simulink model "Non_linear_model_impulse_response"  (R2021b)
settings: Solver=FixedStepAuto  StartTime=0.0  StopTime=30  FixedStep=0.001  RelTol=1e-3  EnableMultiTasking=on
values from neighbouring files (symbols this model uses):
  F = 1.5    [Initial_data.m]
  F_j = 2.7    [Initial_data.m]
  F_js = 1.5    [Initial_data.m]
  F_s = 1    [Initial_data.m]
  T_i = 57    [Initial_data.m]
  T_is = 50    [Initial_data.m]
  T_ji = 206    [Initial_data.m]
  T_jis = 200    [Initial_data.m]
  T_js = 150    [Initial_data.m]
  T_s = 125    [Initial_data.m]
settings Model: Creator=Administrator  LastModifiedBy=Administrator

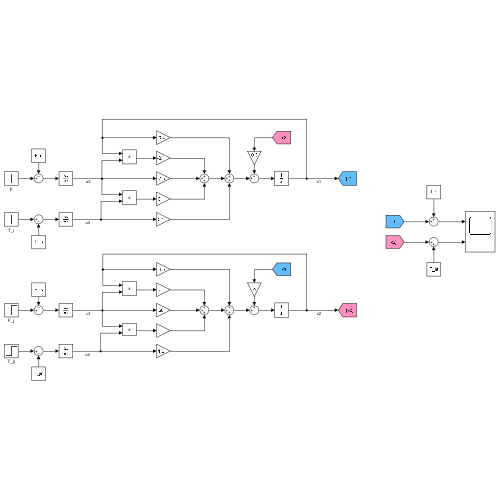
[thumbnail: Simulink's stored preview of the top-level diagram]
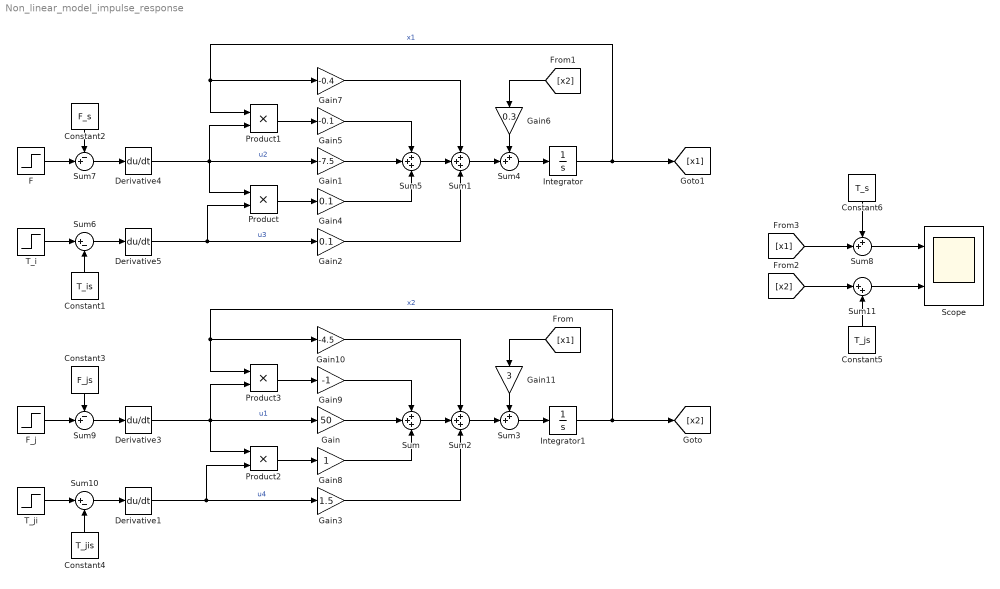
== system Non_linear_model_impulse_response ==
  Constant1 : Constant  Value=T_is
  Constant2 : Constant  Value=F_s
  Constant3 : Constant  Value=F_js
  Constant4 : Constant  Value=T_jis
  Constant5 : Constant  Value=T_js
  Constant6 : Constant  Value=T_s
  Derivative{1,3..5} (4 alike) : Derivative
  F : Step  Time=0.001  After=F  SampleTime=0
  F_j : Step  Time=0.001  After=F_j  SampleTime=0
  Gain : Gain  Gain=50
  Gain1 : Gain  Gain=-7.5
  Gain10 : Gain  Gain=-4.5
  Gain11 : Gain  Gain=3
  Gain2 : Gain  Gain=0.1
  Gain3 : Gain  Gain=1.5
  Gain4 : Gain  Gain=0.1
  Gain5 : Gain  Gain=-0.1
  Gain6 : Gain  Gain=0.3
  Gain7 : Gain  Gain=-0.4
  Gain8 : Gain
  Gain9 : Gain  Gain=-1
  Integrator : Integrator
  Integrator1 : Integrator
  Product{,1..3} (4 alike) : Product
  Scope : Scope  NumInputPorts=2
  Sum{,1..2,5} (4 alike) : Sum  Inputs=+++
  Sum10 : Sum  Inputs=|+-
  Sum11 : Sum  Inputs=|++
  Sum3 : Sum  Inputs=++|
  Sum4 : Sum  Inputs=++|
  Sum6 : Sum  Inputs=|+-
  Sum7 : Sum  Inputs=-+|
  Sum8 : Sum  Inputs=++|
  Sum9 : Sum  Inputs=-+|
  T_i : Step  Time=0.001  After=T_i  SampleTime=0
  T_ji : Step  Time=0.001  After=T_ji  SampleTime=0
  wires:
  Gain/1 -> Sum/2
  Gain2/1 -> Sum1/3
  Gain3/1 -> Sum2/3
  Product/1 -> Gain4/1
  Integrator/1 -> Product1/1, Gain7/1, [x1]  "x1"
  Product1/1 -> Gain5/1
  Gain4/1 -> Sum5/3
  Gain5/1 -> Sum5/1
  Integrator1/1 -> Product3/1, Gain10/1, [x2]  "x2"
  Gain1/1 -> Sum5/2
  Sum5/1 -> Sum1/2
  Gain6/1 -> Sum4/1
  Sum1/1 -> Sum4/2
  Gain7/1 -> Sum1/1
  Sum4/1 -> Integrator/1
  Product2/1 -> Gain8/1
  Sum/1 -> Sum2/2
  Gain8/1 -> Sum/3
  Product3/1 -> Gain9/1
  Gain9/1 -> Sum/1
  Gain10/1 -> Sum2/1
  Sum2/1 -> Sum3/2
  Sum3/1 -> Integrator1/1
  Gain11/1 -> Sum3/1
  [x1] -> Gain11/1
  [x2] -> Gain6/1
  [x1] -> Sum8/2
  Constant1/1 -> Sum6/2
  Constant2/1 -> Sum7/1
  Constant3/1 -> Sum9/1
  Constant4/1 -> Sum10/2
  Sum8/1 -> Scope/1
  Sum11/1 -> Scope/2
  [x2] -> Sum11/1
  Constant5/1 -> Sum11/2
  Constant6/1 -> Sum8/1
  Sum6/1 -> Derivative5/1
  Sum7/1 -> Derivative4/1
  Sum10/1 -> Derivative1/1
  Sum9/1 -> Derivative3/1
  F/1 -> Sum7/2
  T_i/1 -> Sum6/1
  F_j/1 -> Sum9/2
  T_ji/1 -> Sum10/1
  Derivative4/1 -> Product/1, Gain1/1, Product1/2  "u2"
  Derivative5/1 -> Product/2, Gain2/1  "u3"
  Derivative3/1 -> Product2/1, Product3/2, Gain/1  "u1"
  Derivative1/1 -> Product2/2, Gain3/1  "u4"
